simulink model "MG_sim"  (R2020a)
settings: Solver=VariableStepAuto  StartTime=0.0  StopTime=Inf  FixedStep=N*T  RelTol=1e-3
PostLoadFcn:
  | , if any(exist('dsrtsu_mdlpostloadfcn', 'file') ~= 0), dsrtsu_mdlpostloadfcn('Execute', bdroot); end,
InitFcn:
  | , if any(exist('rtifpga_mdlclblib', 'file') ~= 0), rtifpga_mdlclblib('Init', bdroot); end,
model workspace (MAT data in the model file):
  FPGA_MG_sim_1_Register_1_1_1_write : Simulink.Signal (value not decoded)
  FPGA_MG_sim_1_Register_2_1_1_write : Simulink.Signal (value not decoded)
  FPGA_MG_sim_1_Register_3_1_1_write : Simulink.Signal (value not decoded)
values from neighbouring files (symbols this model uses):
  amp = 1    [param.m]
  fixedgain_i = 10*1000/(3*100)    (= 33.3333333333)    [param.m]
  fixedgain_vc1 = 10*10000/(3*100*2.5)    (= 133.333333333)    [param.m]
  fixedgain_vc5 = 10*22000/(3*100*2.5)    (= 293.333333333)    [param.m]
  fixedgain_vdc = 10*22000/(3*100*2.5)    (= 293.333333333)    [param.m]
  freq = 50    [param.m]
  gain_iL1 = 1    [param.m]
  gain_iL2 = 1    [param.m]
  gain_iL3 = 1    [param.m]
  gain_iL4 = 1    [param.m]
  gain_vc1 = 1    [param.m]
  gain_vc5 = 1    [param.m]
  gain_vdc = 1    [param.m]
  Ii = 10    [param.m]
  Ipv = 0.01    [param.m]
  Iv = 0.1    [param.m]
  Ki = 1e-7    (= 1e-07)    [param.m]
  Kp = 0.5    [param.m]
  M = 10    [param.m]
  maxd = N-1    (= 39)    [param.m]
  mind = 1    [param.m]
  N = 40    [param.m]
  offset_iL1 = .2    (= 0.2)    [param.m]
  offset_iL2 = 0.2    [param.m]
  offset_iL3 = 0.3    [param.m]
  offset_iL4 = 0.25    [param.m]
  offset_vc1 = 0.27    [param.m]
  offset_vc5 = 1.3    [param.m]
  offset_vdc = 1.5    [param.m]
  Pi = 0.3    [param.m]
  Ppv = 0.05    [param.m]
  Pv = 0.05    [param.m]
  T = 6e-6    (= 6e-06)    [param.m]
  Tf = 1/1000    (= 0.001)    [param.m]
  Tfdc = 1/20    (= 0.05)    [param.m]
  v_dc_ref = 80    [param.m]
undefined symbols (not defined in the file or in its folder): DiscIntNeverNeededParam
libraries: xbsIndex_r4 x156, rti1202lib_adc_class1 x7, rtiproclib x7, simulink x6, rti1202lib_dac_class1 x1, rtifpgainterfacelib x1
(part 4 of 5)

== system MG_sim/RTI Data/RTI Data Store ==
  RTI Data Store : Subsystem  mask(RTI_DATA_STORE){}
      mask help:
      | RTI Data Store Block. This block is used by RTI to store internal model dependent data. Deleting this block will result in data loss.
      |
      | NEVER DELETE, COPY, OR MODIFY THIS BLOCK!
      mask Help:
      | RTI Data Store Block. This block is used by RTI to store internal model dependent data. Deleting this block will result in data loss.
      | 
      | NEVER DELETE, COPY, OR MODIFY THIS BLOCK!
      mask Display: text(0.5, 0.5, ' ', 'HorizontalAlignment', 'center');

== system MG_sim/fpga/FPGA_INT_BL1 ==
  Int : Inport
  CEP1 : xbsIndex_r4/Clock Enable Probe  inherit_constraints=off  block_type=ceprobe
      settings: infoedit="Clock enable extractor.  Produces a Boolean output that mirrors the hardware clock enable associated with the input sample rate.<br><br>Hardware notes: in hardware this block costs nothing."
  Constant1 : xbsIndex_r4/Constant  const=1  gui_display_data_type=Fixed-point  arith_type=Boolean  n_bits=16  bin_pt=14  preci_type=Single  exp_width=8  frac_width=24  explicit_period=on  period=1*1e-08  equ=P=C  opselect=C  inp2=PCIN>>17  opr=+  inp1=P  carry=CIN  dbl_ovrd=off  block_type=constant
  Convert1 : xbsIndex_r4/Convert  gui_display_data_type=Fixed-point  arith_type=Unsigned  n_bits=1  bin_pt=0  float_type=Single  exp_bits=8  fraction_bits=24  quantization=Truncate  overflow=Wrap  en=off  latency=0  pipeline=off  dbl_ovrd=off  block_type=convert
  Register1 : xbsIndex_r4/Register  init=0  rst=off  en=on  dbl_ovrd=off  block_type=register
  Terminator : Terminator
  phs_interrupt : Subsystem
  usr_interrupt_02 : xbsIndex_r4/Gateway Out  inherit_from_input=off  hdl_port=on  rows=1  columns=1  UseAsDAC=off  DACChannel='1'  interface=None  automatic_assignment=on  address_offset=hex2dec('00')  intf_name=''  intf_description=''  timing_constraint=None  locs_specified=off  LOCs={}  io_standard={}  block_type=gatewayout
  tag scope: FPGA_MG_sim_rtiFPGAtmp_1_Interrupt_3_1_write=global
  wires:
  phs_interrupt/1(data_o) -> [FPGA_MG_sim_rtiFPGAtmp_1_Interrupt_3_1_write], Terminator/1
  usr_interrupt_02/1 -> phs_interrupt/1(data_i)
  Convert1/1 -> Register1/1
  Int/1 -> Convert1/1
  Register1/1 -> usr_interrupt_02/1
  CEP1/1 -> Register1/2
  Constant1/1 -> CEP1/1

== system MG_sim/fpga/FPGA_INT_BL2 ==
  Int : Inport
  CEP1 : xbsIndex_r4/Clock Enable Probe  inherit_constraints=off  block_type=ceprobe
      settings: infoedit="Clock enable extractor.  Produces a Boolean output that mirrors the hardware clock enable associated with the input sample rate.<br><br>Hardware notes: in hardware this block costs nothing."
  Constant1 : xbsIndex_r4/Constant  const=1  gui_display_data_type=Fixed-point  arith_type=Boolean  n_bits=16  bin_pt=14  preci_type=Single  exp_width=8  frac_width=24  explicit_period=on  period=1*1e-08  equ=P=C  opselect=C  inp2=PCIN>>17  opr=+  inp1=P  carry=CIN  dbl_ovrd=off  block_type=constant
  Convert1 : xbsIndex_r4/Convert  gui_display_data_type=Fixed-point  arith_type=Unsigned  n_bits=1  bin_pt=0  float_type=Single  exp_bits=8  fraction_bits=24  quantization=Truncate  overflow=Wrap  en=off  latency=0  pipeline=off  dbl_ovrd=off  block_type=convert
  Register1 : xbsIndex_r4/Register  init=0  rst=off  en=on  dbl_ovrd=off  block_type=register
  Terminator : Terminator
  phs_interrupt : Subsystem
  usr_interrupt_01 : xbsIndex_r4/Gateway Out  inherit_from_input=off  hdl_port=on  rows=1  columns=1  UseAsDAC=off  DACChannel='1'  interface=None  automatic_assignment=on  address_offset=hex2dec('00')  intf_name=''  intf_description=''  timing_constraint=None  locs_specified=off  LOCs={}  io_standard={}  block_type=gatewayout
  tag scope: FPGA_MG_sim_rtiFPGAtmp_1_Interrupt_2_1_write=global
  wires:
  phs_interrupt/1(data_o) -> [FPGA_MG_sim_rtiFPGAtmp_1_Interrupt_2_1_write], Terminator/1
  usr_interrupt_01/1 -> phs_interrupt/1(data_i)
  Convert1/1 -> Register1/1
  Int/1 -> Convert1/1
  Register1/1 -> usr_interrupt_01/1
  CEP1/1 -> Register1/2
  Constant1/1 -> CEP1/1

== system MG_sim/fpga/FPGA_INT_BL3 ==
  Int : Inport
  CEP1 : xbsIndex_r4/Clock Enable Probe  inherit_constraints=off  block_type=ceprobe
      settings: infoedit="Clock enable extractor.  Produces a Boolean output that mirrors the hardware clock enable associated with the input sample rate.<br><br>Hardware notes: in hardware this block costs nothing."
  Constant1 : xbsIndex_r4/Constant  const=1  gui_display_data_type=Fixed-point  arith_type=Boolean  n_bits=16  bin_pt=14  preci_type=Single  exp_width=8  frac_width=24  explicit_period=on  period=1*1e-08  equ=P=C  opselect=C  inp2=PCIN>>17  opr=+  inp1=P  carry=CIN  dbl_ovrd=off  block_type=constant
  Convert1 : xbsIndex_r4/Convert  gui_display_data_type=Fixed-point  arith_type=Unsigned  n_bits=1  bin_pt=0  float_type=Single  exp_bits=8  fraction_bits=24  quantization=Truncate  overflow=Wrap  en=off  latency=0  pipeline=off  dbl_ovrd=off  block_type=convert
  Register1 : xbsIndex_r4/Register  init=0  rst=off  en=on  dbl_ovrd=off  block_type=register
  Terminator : Terminator
  phs_interrupt : Subsystem
  usr_interrupt_00 : xbsIndex_r4/Gateway Out  inherit_from_input=off  hdl_port=on  rows=1  columns=1  UseAsDAC=off  DACChannel='1'  interface=None  automatic_assignment=on  address_offset=hex2dec('00')  intf_name=''  intf_description=''  timing_constraint=None  locs_specified=off  LOCs={}  io_standard={}  block_type=gatewayout
  tag scope: FPGA_MG_sim_rtiFPGAtmp_1_Interrupt_1_1_write=global
  wires:
  phs_interrupt/1(data_o) -> [FPGA_MG_sim_rtiFPGAtmp_1_Interrupt_1_1_write], Terminator/1
  usr_interrupt_00/1 -> phs_interrupt/1(data_i)
  Convert1/1 -> Register1/1
  Int/1 -> Convert1/1
  Register1/1 -> usr_interrupt_00/1
  CEP1/1 -> Register1/2
  Constant1/1 -> CEP1/1

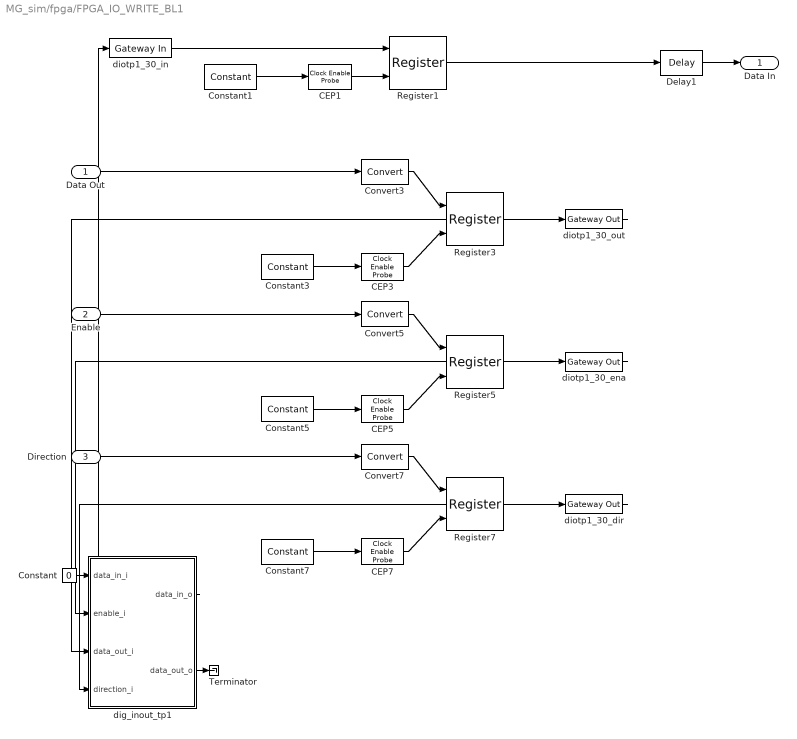
== system MG_sim/fpga/FPGA_IO_WRITE_BL1 ==
  Data Out : Inport
  Enable : Inport  Port=2
  Direction : Inport  Port=3
  CEP{1,3,5,7} (4 alike) : xbsIndex_r4/Clock Enable Probe  inherit_constraints=off  block_type=ceprobe
      settings: infoedit="Clock enable extractor.  Produces a Boolean output that mirrors the hardware clock enable associated with the input sample rate.<br><br>Hardware notes: in hardware this block costs nothing."
  Constant : Constant  Value=0
  Constant{1,3,5,7} (4 alike) : xbsIndex_r4/Constant  const=1  gui_display_data_type=Fixed-point  arith_type=Boolean  n_bits=16  bin_pt=14  preci_type=Single  exp_width=8  frac_width=24  explicit_period=on  period=1*1e-08  equ=P=C  opselect=C  inp2=PCIN>>17  opr=+  inp1=P  carry=CIN  dbl_ovrd=off  block_type=constant
  Convert3 : xbsIndex_r4/Convert  gui_display_data_type=Fixed-point  arith_type=Unsigned  n_bits=1  bin_pt=0  float_type=Single  exp_bits=8  fraction_bits=24  quantization=Truncate  overflow=Wrap  en=off  latency=0  pipeline=off  dbl_ovrd=off  block_type=convert
  Convert5 : xbsIndex_r4/Convert  gui_display_data_type=Fixed-point  arith_type=Unsigned  n_bits=1  bin_pt=0  float_type=Single  exp_bits=8  fraction_bits=24  quantization=Truncate  overflow=Wrap  en=off  latency=0  pipeline=off  dbl_ovrd=off  block_type=convert
  Convert7 : xbsIndex_r4/Convert  gui_display_data_type=Fixed-point  arith_type=Unsigned  n_bits=1  bin_pt=0  float_type=Single  exp_bits=8  fraction_bits=24  quantization=Truncate  overflow=Wrap  en=off  latency=0  pipeline=off  dbl_ovrd=off  block_type=convert
  Delay1 : xbsIndex_r4/Delay  rst=off  infoeditControl=Selection of Reset will increase slice count due to use of real FFs and instead of SRLs  en=off  latency=0  reg_retiming=off  dbl_ovrd=off  block_type=delay
  Register{1,3,5,7} (4 alike) : xbsIndex_r4/Register  init=0  rst=off  en=on  dbl_ovrd=off  block_type=register
  Terminator : Terminator
  dig_inout_tp1 : Subsystem
      mask init:
      | par = rtifpgafcnlib('GetCurrentParaValue', get_param(get(gcbh, 'parent'), 'handle'));
      | if isempty(par)
      |     return
      | end
      | inverted_dio = str2double(par(2).Value{1});
      | vsetting = str2double(par(5).Value{1});
      | switch vsetting 
      |     case 1
      |         voltage = 3.3
      |     case 2
      |         voltage = 2.5;
      |     otherwise
      |         voltage = 5;
      | end
  diotp1_30_dir : xbsIndex_r4/Gateway Out  inherit_from_input=off  hdl_port=on  rows=1  columns=1  UseAsDAC=off  DACChannel='1'  interface=None  automatic_assignment=on  address_offset=hex2dec('00')  intf_name=''  intf_description=''  timing_constraint=None  locs_specified=off  LOCs={}  io_standard={}  block_type=gatewayout
  diotp1_30_ena : xbsIndex_r4/Gateway Out  inherit_from_input=off  hdl_port=on  rows=1  columns=1  UseAsDAC=off  DACChannel='1'  interface=None  automatic_assignment=on  address_offset=hex2dec('00')  intf_name=''  intf_description=''  timing_constraint=None  locs_specified=off  LOCs={}  io_standard={}  block_type=gatewayout
  diotp1_30_in : xbsIndex_r4/Gateway In  gui_display_data_type=Fixed-point  arith_type=Unsigned  n_bits=1  bin_pt=0  preci_type=Single  exp_width=8  frac_width=24  rows=1  columns=1  quantization="Round  (unbiased: +/- Inf)"  overflow=Saturate  period=1e-08  UseAsADC=off  ADCChannel='1'  interface=None  automatic_assignment=on  address_offset=hex2dec('00')  intf_name=''  intf_description=''  default_value=0  timing_constraint=None  locs_specified=off  LOCs={}  io_standard={}  inherit_from_input=off  hdl_port=on  dbl_ovrd=off  block_type=gatewayin
  diotp1_30_out : xbsIndex_r4/Gateway Out  inherit_from_input=off  hdl_port=on  rows=1  columns=1  UseAsDAC=off  DACChannel='1'  interface=None  automatic_assignment=on  address_offset=hex2dec('00')  intf_name=''  intf_description=''  timing_constraint=None  locs_specified=off  LOCs={}  io_standard={}  block_type=gatewayout
  Data In : Outport
  wires:
  dig_inout_tp1/2(data_out_o) -> Terminator/1
  Constant/1 -> dig_inout_tp1/1(data_in_i)
  diotp1_30_dir/1 -> dig_inout_tp1/4(direction_i)
  diotp1_30_ena/1 -> dig_inout_tp1/2(enable_i)
  diotp1_30_out/1 -> dig_inout_tp1/3(data_out_i)
  dig_inout_tp1/1(data_in_o) -> diotp1_30_in/1
  Convert7/1 -> Register7/1
  Direction/1 -> Convert7/1
  Register7/1 -> diotp1_30_dir/1
  CEP7/1 -> Register7/2
  Constant7/1 -> CEP7/1
  Convert5/1 -> Register5/1
  Enable/1 -> Convert5/1
  Register5/1 -> diotp1_30_ena/1
  CEP5/1 -> Register5/2
  Constant5/1 -> CEP5/1
  Convert3/1 -> Register3/1
  Data Out/1 -> Convert3/1
  Register3/1 -> diotp1_30_out/1
  CEP3/1 -> Register3/2
  Constant3/1 -> CEP3/1
  diotp1_30_in/1 -> Register1/1
  CEP1/1 -> Register1/2
  Constant1/1 -> CEP1/1
  Delay1/1 -> Data In/1
  Register1/1 -> Delay1/1

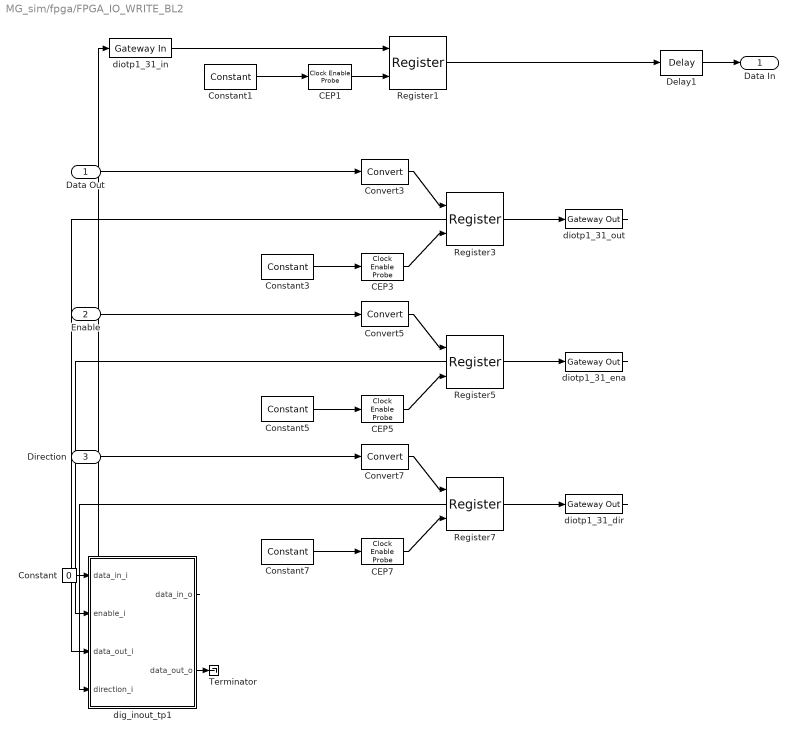
== system MG_sim/fpga/FPGA_IO_WRITE_BL2 ==
  Data Out : Inport
  Enable : Inport  Port=2
  Direction : Inport  Port=3
  CEP{1,3,5,7} (4 alike) : xbsIndex_r4/Clock Enable Probe  inherit_constraints=off  block_type=ceprobe
      settings: infoedit="Clock enable extractor.  Produces a Boolean output that mirrors the hardware clock enable associated with the input sample rate.<br><br>Hardware notes: in hardware this block costs nothing."
  Constant : Constant  Value=0
  Constant{1,3,5,7} (4 alike) : xbsIndex_r4/Constant  const=1  gui_display_data_type=Fixed-point  arith_type=Boolean  n_bits=16  bin_pt=14  preci_type=Single  exp_width=8  frac_width=24  explicit_period=on  period=1*1e-08  equ=P=C  opselect=C  inp2=PCIN>>17  opr=+  inp1=P  carry=CIN  dbl_ovrd=off  block_type=constant
  Convert3 : xbsIndex_r4/Convert  gui_display_data_type=Fixed-point  arith_type=Unsigned  n_bits=1  bin_pt=0  float_type=Single  exp_bits=8  fraction_bits=24  quantization=Truncate  overflow=Wrap  en=off  latency=0  pipeline=off  dbl_ovrd=off  block_type=convert
  Convert5 : xbsIndex_r4/Convert  gui_display_data_type=Fixed-point  arith_type=Unsigned  n_bits=1  bin_pt=0  float_type=Single  exp_bits=8  fraction_bits=24  quantization=Truncate  overflow=Wrap  en=off  latency=0  pipeline=off  dbl_ovrd=off  block_type=convert
  Convert7 : xbsIndex_r4/Convert  gui_display_data_type=Fixed-point  arith_type=Unsigned  n_bits=1  bin_pt=0  float_type=Single  exp_bits=8  fraction_bits=24  quantization=Truncate  overflow=Wrap  en=off  latency=0  pipeline=off  dbl_ovrd=off  block_type=convert
  Delay1 : xbsIndex_r4/Delay  rst=off  infoeditControl=Selection of Reset will increase slice count due to use of real FFs and instead of SRLs  en=off  latency=0  reg_retiming=off  dbl_ovrd=off  block_type=delay
  Register{1,3,5,7} (4 alike) : xbsIndex_r4/Register  init=0  rst=off  en=on  dbl_ovrd=off  block_type=register
  Terminator : Terminator
  dig_inout_tp1 : Subsystem
      mask init: same as MG_sim/fpga/FPGA_IO_WRITE_BL1/dig_inout_tp1
  diotp1_31_dir : xbsIndex_r4/Gateway Out  inherit_from_input=off  hdl_port=on  rows=1  columns=1  UseAsDAC=off  DACChannel='1'  interface=None  automatic_assignment=on  address_offset=hex2dec('00')  intf_name=''  intf_description=''  timing_constraint=None  locs_specified=off  LOCs={}  io_standard={}  block_type=gatewayout
  diotp1_31_ena : xbsIndex_r4/Gateway Out  inherit_from_input=off  hdl_port=on  rows=1  columns=1  UseAsDAC=off  DACChannel='1'  interface=None  automatic_assignment=on  address_offset=hex2dec('00')  intf_name=''  intf_description=''  timing_constraint=None  locs_specified=off  LOCs={}  io_standard={}  block_type=gatewayout
  diotp1_31_in : xbsIndex_r4/Gateway In  gui_display_data_type=Fixed-point  arith_type=Unsigned  n_bits=1  bin_pt=0  preci_type=Single  exp_width=8  frac_width=24  rows=1  columns=1  quantization="Round  (unbiased: +/- Inf)"  overflow=Saturate  period=1e-08  UseAsADC=off  ADCChannel='1'  interface=None  automatic_assignment=on  address_offset=hex2dec('00')  intf_name=''  intf_description=''  default_value=0  timing_constraint=None  locs_specified=off  LOCs={}  io_standard={}  inherit_from_input=off  hdl_port=on  dbl_ovrd=off  block_type=gatewayin
  diotp1_31_out : xbsIndex_r4/Gateway Out  inherit_from_input=off  hdl_port=on  rows=1  columns=1  UseAsDAC=off  DACChannel='1'  interface=None  automatic_assignment=on  address_offset=hex2dec('00')  intf_name=''  intf_description=''  timing_constraint=None  locs_specified=off  LOCs={}  io_standard={}  block_type=gatewayout
  Data In : Outport
  wires:
  dig_inout_tp1/2(data_out_o) -> Terminator/1
  Constant/1 -> dig_inout_tp1/1(data_in_i)
  diotp1_31_dir/1 -> dig_inout_tp1/4(direction_i)
  diotp1_31_ena/1 -> dig_inout_tp1/2(enable_i)
  diotp1_31_out/1 -> dig_inout_tp1/3(data_out_i)
  dig_inout_tp1/1(data_in_o) -> diotp1_31_in/1
  Convert7/1 -> Register7/1
  Direction/1 -> Convert7/1
  Register7/1 -> diotp1_31_dir/1
  CEP7/1 -> Register7/2
  Constant7/1 -> CEP7/1
  Convert5/1 -> Register5/1
  Enable/1 -> Convert5/1
  Register5/1 -> diotp1_31_ena/1
  CEP5/1 -> Register5/2
  Constant5/1 -> CEP5/1
  Convert3/1 -> Register3/1
  Data Out/1 -> Convert3/1
  Register3/1 -> diotp1_31_out/1
  CEP3/1 -> Register3/2
  Constant3/1 -> CEP3/1
  diotp1_31_in/1 -> Register1/1
  CEP1/1 -> Register1/2
  Constant1/1 -> CEP1/1
  Delay1/1 -> Data In/1
  Register1/1 -> Delay1/1

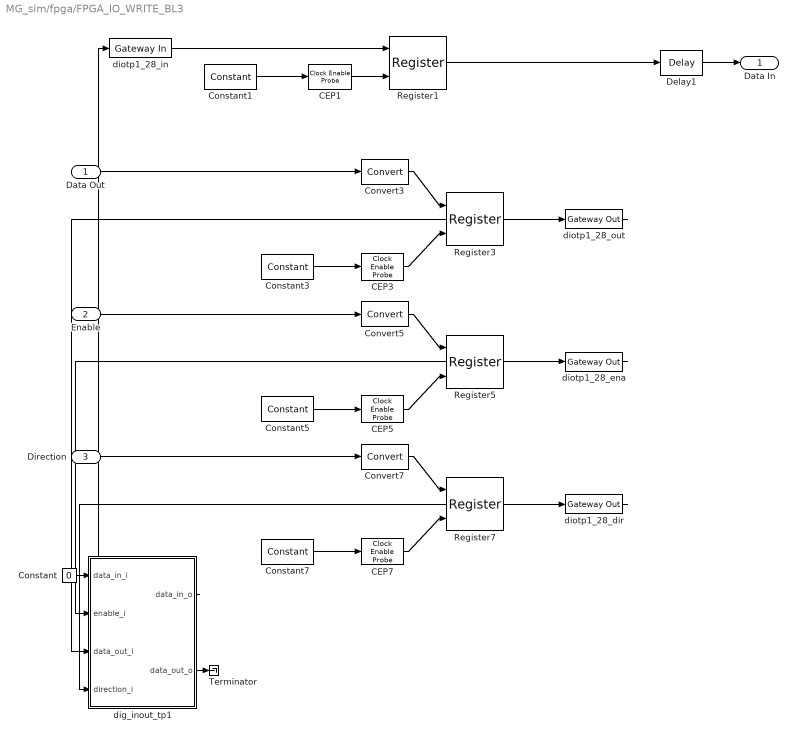
== system MG_sim/fpga/FPGA_IO_WRITE_BL3 ==
  Data Out : Inport
  Enable : Inport  Port=2
  Direction : Inport  Port=3
  CEP{1,3,5,7} (4 alike) : xbsIndex_r4/Clock Enable Probe  inherit_constraints=off  block_type=ceprobe
      settings: infoedit="Clock enable extractor.  Produces a Boolean output that mirrors the hardware clock enable associated with the input sample rate.<br><br>Hardware notes: in hardware this block costs nothing."
  Constant : Constant  Value=0
  Constant{1,3,5,7} (4 alike) : xbsIndex_r4/Constant  const=1  gui_display_data_type=Fixed-point  arith_type=Boolean  n_bits=16  bin_pt=14  preci_type=Single  exp_width=8  frac_width=24  explicit_period=on  period=1*1e-08  equ=P=C  opselect=C  inp2=PCIN>>17  opr=+  inp1=P  carry=CIN  dbl_ovrd=off  block_type=constant
  Convert3 : xbsIndex_r4/Convert  gui_display_data_type=Fixed-point  arith_type=Unsigned  n_bits=1  bin_pt=0  float_type=Single  exp_bits=8  fraction_bits=24  quantization=Truncate  overflow=Wrap  en=off  latency=0  pipeline=off  dbl_ovrd=off  block_type=convert
  Convert5 : xbsIndex_r4/Convert  gui_display_data_type=Fixed-point  arith_type=Unsigned  n_bits=1  bin_pt=0  float_type=Single  exp_bits=8  fraction_bits=24  quantization=Truncate  overflow=Wrap  en=off  latency=0  pipeline=off  dbl_ovrd=off  block_type=convert
  Convert7 : xbsIndex_r4/Convert  gui_display_data_type=Fixed-point  arith_type=Unsigned  n_bits=1  bin_pt=0  float_type=Single  exp_bits=8  fraction_bits=24  quantization=Truncate  overflow=Wrap  en=off  latency=0  pipeline=off  dbl_ovrd=off  block_type=convert
  Delay1 : xbsIndex_r4/Delay  rst=off  infoeditControl=Selection of Reset will increase slice count due to use of real FFs and instead of SRLs  en=off  latency=0  reg_retiming=off  dbl_ovrd=off  block_type=delay
  Register{1,3,5,7} (4 alike) : xbsIndex_r4/Register  init=0  rst=off  en=on  dbl_ovrd=off  block_type=register
  Terminator : Terminator
  dig_inout_tp1 : Subsystem
      mask init: same as MG_sim/fpga/FPGA_IO_WRITE_BL1/dig_inout_tp1
  diotp1_28_dir : xbsIndex_r4/Gateway Out  inherit_from_input=off  hdl_port=on  rows=1  columns=1  UseAsDAC=off  DACChannel='1'  interface=None  automatic_assignment=on  address_offset=hex2dec('00')  intf_name=''  intf_description=''  timing_constraint=None  locs_specified=off  LOCs={}  io_standard={}  block_type=gatewayout
  diotp1_28_ena : xbsIndex_r4/Gateway Out  inherit_from_input=off  hdl_port=on  rows=1  columns=1  UseAsDAC=off  DACChannel='1'  interface=None  automatic_assignment=on  address_offset=hex2dec('00')  intf_name=''  intf_description=''  timing_constraint=None  locs_specified=off  LOCs={}  io_standard={}  block_type=gatewayout
  diotp1_28_in : xbsIndex_r4/Gateway In  gui_display_data_type=Fixed-point  arith_type=Unsigned  n_bits=1  bin_pt=0  preci_type=Single  exp_width=8  frac_width=24  rows=1  columns=1  quantization="Round  (unbiased: +/- Inf)"  overflow=Saturate  period=1e-08  UseAsADC=off  ADCChannel='1'  interface=None  automatic_assignment=on  address_offset=hex2dec('00')  intf_name=''  intf_description=''  default_value=0  timing_constraint=None  locs_specified=off  LOCs={}  io_standard={}  inherit_from_input=off  hdl_port=on  dbl_ovrd=off  block_type=gatewayin
  diotp1_28_out : xbsIndex_r4/Gateway Out  inherit_from_input=off  hdl_port=on  rows=1  columns=1  UseAsDAC=off  DACChannel='1'  interface=None  automatic_assignment=on  address_offset=hex2dec('00')  intf_name=''  intf_description=''  timing_constraint=None  locs_specified=off  LOCs={}  io_standard={}  block_type=gatewayout
  Data In : Outport
  wires:
  dig_inout_tp1/2(data_out_o) -> Terminator/1
  Constant/1 -> dig_inout_tp1/1(data_in_i)
  diotp1_28_dir/1 -> dig_inout_tp1/4(direction_i)
  diotp1_28_ena/1 -> dig_inout_tp1/2(enable_i)
  diotp1_28_out/1 -> dig_inout_tp1/3(data_out_i)
  dig_inout_tp1/1(data_in_o) -> diotp1_28_in/1
  Convert7/1 -> Register7/1
  Direction/1 -> Convert7/1
  Register7/1 -> diotp1_28_dir/1
  CEP7/1 -> Register7/2
  Constant7/1 -> CEP7/1
  Convert5/1 -> Register5/1
  Enable/1 -> Convert5/1
  Register5/1 -> diotp1_28_ena/1
  CEP5/1 -> Register5/2
  Constant5/1 -> CEP5/1
  Convert3/1 -> Register3/1
  Data Out/1 -> Convert3/1
  Register3/1 -> diotp1_28_out/1
  CEP3/1 -> Register3/2
  Constant3/1 -> CEP3/1
  diotp1_28_in/1 -> Register1/1
  CEP1/1 -> Register1/2
  Constant1/1 -> CEP1/1
  Delay1/1 -> Data In/1
  Register1/1 -> Delay1/1

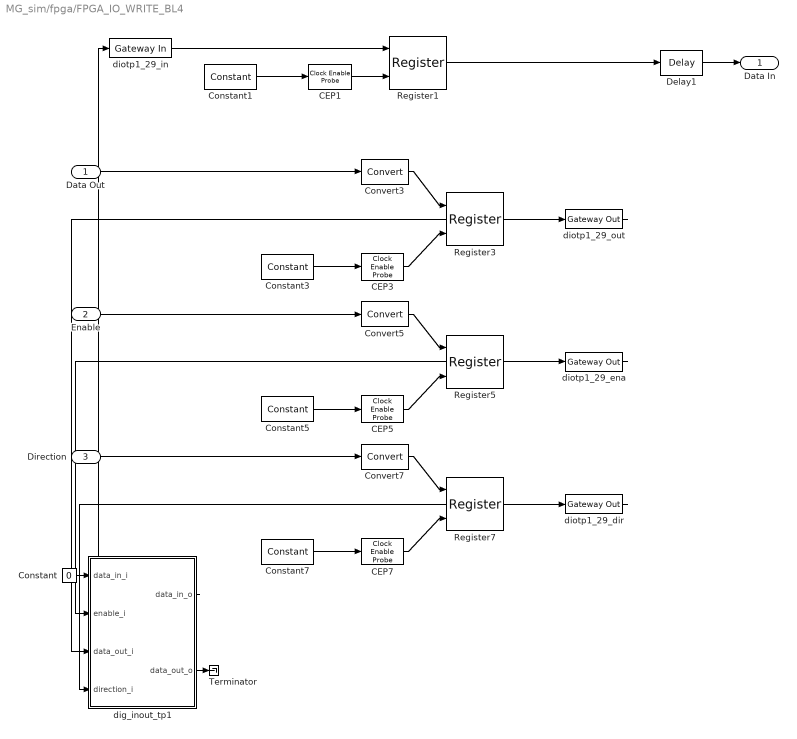
== system MG_sim/fpga/FPGA_IO_WRITE_BL4 ==
  Data Out : Inport
  Enable : Inport  Port=2
  Direction : Inport  Port=3
  CEP{1,3,5,7} (4 alike) : xbsIndex_r4/Clock Enable Probe  inherit_constraints=off  block_type=ceprobe
      settings: infoedit="Clock enable extractor.  Produces a Boolean output that mirrors the hardware clock enable associated with the input sample rate.<br><br>Hardware notes: in hardware this block costs nothing."
  Constant : Constant  Value=0
  Constant{1,3,5,7} (4 alike) : xbsIndex_r4/Constant  const=1  gui_display_data_type=Fixed-point  arith_type=Boolean  n_bits=16  bin_pt=14  preci_type=Single  exp_width=8  frac_width=24  explicit_period=on  period=1*1e-08  equ=P=C  opselect=C  inp2=PCIN>>17  opr=+  inp1=P  carry=CIN  dbl_ovrd=off  block_type=constant
  Convert3 : xbsIndex_r4/Convert  gui_display_data_type=Fixed-point  arith_type=Unsigned  n_bits=1  bin_pt=0  float_type=Single  exp_bits=8  fraction_bits=24  quantization=Truncate  overflow=Wrap  en=off  latency=0  pipeline=off  dbl_ovrd=off  block_type=convert
  Convert5 : xbsIndex_r4/Convert  gui_display_data_type=Fixed-point  arith_type=Unsigned  n_bits=1  bin_pt=0  float_type=Single  exp_bits=8  fraction_bits=24  quantization=Truncate  overflow=Wrap  en=off  latency=0  pipeline=off  dbl_ovrd=off  block_type=convert
  Convert7 : xbsIndex_r4/Convert  gui_display_data_type=Fixed-point  arith_type=Unsigned  n_bits=1  bin_pt=0  float_type=Single  exp_bits=8  fraction_bits=24  quantization=Truncate  overflow=Wrap  en=off  latency=0  pipeline=off  dbl_ovrd=off  block_type=convert
  Delay1 : xbsIndex_r4/Delay  rst=off  infoeditControl=Selection of Reset will increase slice count due to use of real FFs and instead of SRLs  en=off  latency=0  reg_retiming=off  dbl_ovrd=off  block_type=delay
  Register{1,3,5,7} (4 alike) : xbsIndex_r4/Register  init=0  rst=off  en=on  dbl_ovrd=off  block_type=register
  Terminator : Terminator
  dig_inout_tp1 : Subsystem
      mask init: same as MG_sim/fpga/FPGA_IO_WRITE_BL1/dig_inout_tp1
  diotp1_29_dir : xbsIndex_r4/Gateway Out  inherit_from_input=off  hdl_port=on  rows=1  columns=1  UseAsDAC=off  DACChannel='1'  interface=None  automatic_assignment=on  address_offset=hex2dec('00')  intf_name=''  intf_description=''  timing_constraint=None  locs_specified=off  LOCs={}  io_standard={}  block_type=gatewayout
  diotp1_29_ena : xbsIndex_r4/Gateway Out  inherit_from_input=off  hdl_port=on  rows=1  columns=1  UseAsDAC=off  DACChannel='1'  interface=None  automatic_assignment=on  address_offset=hex2dec('00')  intf_name=''  intf_description=''  timing_constraint=None  locs_specified=off  LOCs={}  io_standard={}  block_type=gatewayout
  diotp1_29_in : xbsIndex_r4/Gateway In  gui_display_data_type=Fixed-point  arith_type=Unsigned  n_bits=1  bin_pt=0  preci_type=Single  exp_width=8  frac_width=24  rows=1  columns=1  quantization="Round  (unbiased: +/- Inf)"  overflow=Saturate  period=1e-08  UseAsADC=off  ADCChannel='1'  interface=None  automatic_assignment=on  address_offset=hex2dec('00')  intf_name=''  intf_description=''  default_value=0  timing_constraint=None  locs_specified=off  LOCs={}  io_standard={}  inherit_from_input=off  hdl_port=on  dbl_ovrd=off  block_type=gatewayin
  diotp1_29_out : xbsIndex_r4/Gateway Out  inherit_from_input=off  hdl_port=on  rows=1  columns=1  UseAsDAC=off  DACChannel='1'  interface=None  automatic_assignment=on  address_offset=hex2dec('00')  intf_name=''  intf_description=''  timing_constraint=None  locs_specified=off  LOCs={}  io_standard={}  block_type=gatewayout
  Data In : Outport
  wires:
  dig_inout_tp1/2(data_out_o) -> Terminator/1
  Constant/1 -> dig_inout_tp1/1(data_in_i)
  diotp1_29_dir/1 -> dig_inout_tp1/4(direction_i)
  diotp1_29_ena/1 -> dig_inout_tp1/2(enable_i)
  diotp1_29_out/1 -> dig_inout_tp1/3(data_out_i)
  dig_inout_tp1/1(data_in_o) -> diotp1_29_in/1
  Convert7/1 -> Register7/1
  Direction/1 -> Convert7/1
  Register7/1 -> diotp1_29_dir/1
  CEP7/1 -> Register7/2
  Constant7/1 -> CEP7/1
  Convert5/1 -> Register5/1
  Enable/1 -> Convert5/1
  Register5/1 -> diotp1_29_ena/1
  CEP5/1 -> Register5/2
  Constant5/1 -> CEP5/1
  Convert3/1 -> Register3/1
  Data Out/1 -> Convert3/1
  Register3/1 -> diotp1_29_out/1
  CEP3/1 -> Register3/2
  Constant3/1 -> CEP3/1
  diotp1_29_in/1 -> Register1/1
  CEP1/1 -> Register1/2
  Constant1/1 -> CEP1/1
  Delay1/1 -> Data In/1
  Register1/1 -> Delay1/1

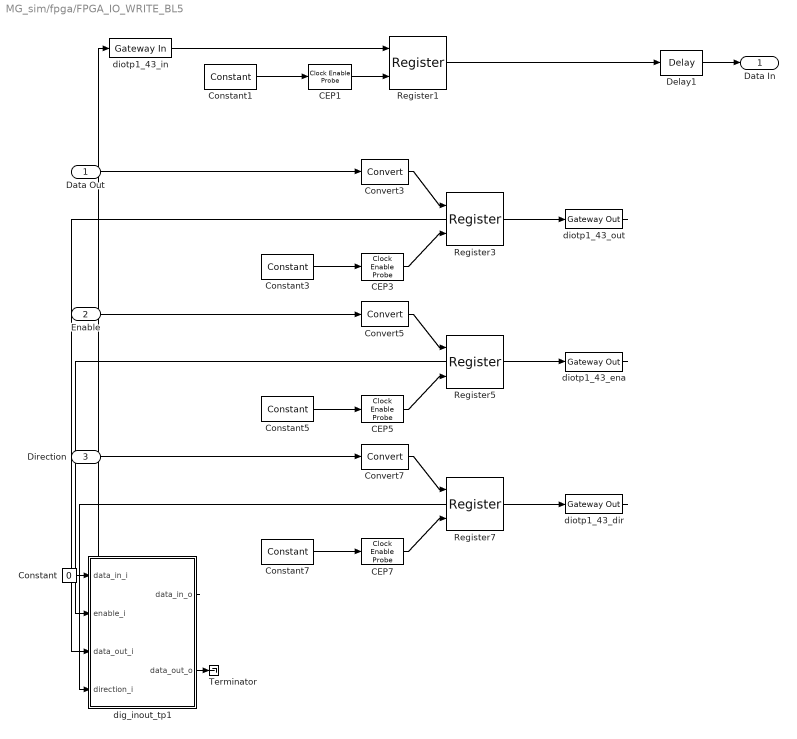
== system MG_sim/fpga/FPGA_IO_WRITE_BL5 ==
  Data Out : Inport
  Enable : Inport  Port=2
  Direction : Inport  Port=3
  CEP{1,3,5,7} (4 alike) : xbsIndex_r4/Clock Enable Probe  inherit_constraints=off  block_type=ceprobe
      settings: infoedit="Clock enable extractor.  Produces a Boolean output that mirrors the hardware clock enable associated with the input sample rate.<br><br>Hardware notes: in hardware this block costs nothing."
  Constant : Constant  Value=0
  Constant{1,3,5,7} (4 alike) : xbsIndex_r4/Constant  const=1  gui_display_data_type=Fixed-point  arith_type=Boolean  n_bits=16  bin_pt=14  preci_type=Single  exp_width=8  frac_width=24  explicit_period=on  period=1*1e-08  equ=P=C  opselect=C  inp2=PCIN>>17  opr=+  inp1=P  carry=CIN  dbl_ovrd=off  block_type=constant
  Convert3 : xbsIndex_r4/Convert  gui_display_data_type=Fixed-point  arith_type=Unsigned  n_bits=1  bin_pt=0  float_type=Single  exp_bits=8  fraction_bits=24  quantization=Truncate  overflow=Wrap  en=off  latency=0  pipeline=off  dbl_ovrd=off  block_type=convert
  Convert5 : xbsIndex_r4/Convert  gui_display_data_type=Fixed-point  arith_type=Unsigned  n_bits=1  bin_pt=0  float_type=Single  exp_bits=8  fraction_bits=24  quantization=Truncate  overflow=Wrap  en=off  latency=0  pipeline=off  dbl_ovrd=off  block_type=convert
  Convert7 : xbsIndex_r4/Convert  gui_display_data_type=Fixed-point  arith_type=Unsigned  n_bits=1  bin_pt=0  float_type=Single  exp_bits=8  fraction_bits=24  quantization=Truncate  overflow=Wrap  en=off  latency=0  pipeline=off  dbl_ovrd=off  block_type=convert
  Delay1 : xbsIndex_r4/Delay  rst=off  infoeditControl=Selection of Reset will increase slice count due to use of real FFs and instead of SRLs  en=off  latency=0  reg_retiming=off  dbl_ovrd=off  block_type=delay
  Register{1,3,5,7} (4 alike) : xbsIndex_r4/Register  init=0  rst=off  en=on  dbl_ovrd=off  block_type=register
  Terminator : Terminator
  dig_inout_tp1 : Subsystem
      mask init: same as MG_sim/fpga/FPGA_IO_WRITE_BL1/dig_inout_tp1
  diotp1_43_dir : xbsIndex_r4/Gateway Out  inherit_from_input=off  hdl_port=on  rows=1  columns=1  UseAsDAC=off  DACChannel='1'  interface=None  automatic_assignment=on  address_offset=hex2dec('00')  intf_name=''  intf_description=''  timing_constraint=None  locs_specified=off  LOCs={}  io_standard={}  block_type=gatewayout
  diotp1_43_ena : xbsIndex_r4/Gateway Out  inherit_from_input=off  hdl_port=on  rows=1  columns=1  UseAsDAC=off  DACChannel='1'  interface=None  automatic_assignment=on  address_offset=hex2dec('00')  intf_name=''  intf_description=''  timing_constraint=None  locs_specified=off  LOCs={}  io_standard={}  block_type=gatewayout
  diotp1_43_in : xbsIndex_r4/Gateway In  gui_display_data_type=Fixed-point  arith_type=Unsigned  n_bits=1  bin_pt=0  preci_type=Single  exp_width=8  frac_width=24  rows=1  columns=1  quantization="Round  (unbiased: +/- Inf)"  overflow=Saturate  period=1e-08  UseAsADC=off  ADCChannel='1'  interface=None  automatic_assignment=on  address_offset=hex2dec('00')  intf_name=''  intf_description=''  default_value=0  timing_constraint=None  locs_specified=off  LOCs={}  io_standard={}  inherit_from_input=off  hdl_port=on  dbl_ovrd=off  block_type=gatewayin
  diotp1_43_out : xbsIndex_r4/Gateway Out  inherit_from_input=off  hdl_port=on  rows=1  columns=1  UseAsDAC=off  DACChannel='1'  interface=None  automatic_assignment=on  address_offset=hex2dec('00')  intf_name=''  intf_description=''  timing_constraint=None  locs_specified=off  LOCs={}  io_standard={}  block_type=gatewayout
  Data In : Outport
  wires:
  dig_inout_tp1/2(data_out_o) -> Terminator/1
  Constant/1 -> dig_inout_tp1/1(data_in_i)
  diotp1_43_dir/1 -> dig_inout_tp1/4(direction_i)
  diotp1_43_ena/1 -> dig_inout_tp1/2(enable_i)
  diotp1_43_out/1 -> dig_inout_tp1/3(data_out_i)
  dig_inout_tp1/1(data_in_o) -> diotp1_43_in/1
  Convert7/1 -> Register7/1
  Direction/1 -> Convert7/1
  Register7/1 -> diotp1_43_dir/1
  CEP7/1 -> Register7/2
  Constant7/1 -> CEP7/1
  Convert5/1 -> Register5/1
  Enable/1 -> Convert5/1
  Register5/1 -> diotp1_43_ena/1
  CEP5/1 -> Register5/2
  Constant5/1 -> CEP5/1
  Convert3/1 -> Register3/1
  Data Out/1 -> Convert3/1
  Register3/1 -> diotp1_43_out/1
  CEP3/1 -> Register3/2
  Constant3/1 -> CEP3/1
  diotp1_43_in/1 -> Register1/1
  CEP1/1 -> Register1/2
  Constant1/1 -> CEP1/1
  Delay1/1 -> Data In/1
  Register1/1 -> Delay1/1

== system MG_sim/fpga/FPGA_XDATA_READ_BL1 ==
  CEP1 : xbsIndex_r4/Clock Enable Probe  inherit_constraints=off  block_type=ceprobe
      settings: infoedit="Clock enable extractor.  Produces a Boolean output that mirrors the hardware clock enable associated with the input sample rate.<br><br>Hardware notes: in hardware this block costs nothing."
  CEP3 : xbsIndex_r4/Clock Enable Probe  inherit_constraints=off  block_type=ceprobe
      settings: infoedit="Clock enable extractor.  Produces a Boolean output that mirrors the hardware clock enable associated with the input sample rate.<br><br>Hardware notes: in hardware this block costs nothing."
  Constant1 : xbsIndex_r4/Constant  const=1  gui_display_data_type=Fixed-point  arith_type=Boolean  n_bits=16  bin_pt=14  preci_type=Single  exp_width=8  frac_width=24  explicit_period=on  period=1*1e-08  equ=P=C  opselect=C  inp2=PCIN>>17  opr=+  inp1=P  carry=CIN  dbl_ovrd=off  block_type=constant
  Constant3 : xbsIndex_r4/Constant  const=1  gui_display_data_type=Fixed-point  arith_type=Boolean  n_bits=16  bin_pt=14  preci_type=Single  exp_width=8  frac_width=24  explicit_period=on  period=1*1e-08  equ=P=C  opselect=C  inp2=PCIN>>17  opr=+  inp1=P  carry=CIN  dbl_ovrd=off  block_type=constant
  Delay1 : xbsIndex_r4/Delay  rst=off  infoeditControl=Selection of Reset will increase slice count due to use of real FFs and instead of SRLs  en=off  latency=0  reg_retiming=off  dbl_ovrd=off  block_type=delay
  Delay3 : xbsIndex_r4/Delay  rst=off  infoeditControl=Selection of Reset will increase slice count due to use of real FFs and instead of SRLs  en=off  latency=0  reg_retiming=off  dbl_ovrd=off  block_type=delay
  Register1 : xbsIndex_r4/Register  init=0  rst=off  en=on  dbl_ovrd=off  block_type=register
  Register3 : xbsIndex_r4/Register  init=0  rst=off  en=on  dbl_ovrd=off  block_type=register
  phs_read_register : Subsystem
      mask init:
      | [par, fct] = rtifpgafcnlib('GetCurrentParaValue', get_param(get(gcbh, 'parent'), 'handle'), 'all');
      | if isempty(par) || isempty(fct)
      |     return
      | end
      | binaryPoint = str2double(par(1).Value{1});
      | format = par(2).Value{1};
      | if (strcmp(format, 'signed') == 1)
      |     mode = 0;
      | elseif (strcmp(format, 'unsigned') == 1)
      |     mode = 1;
      | else
      |     % floating-point
      |     mode = 2;
      | end
      | 
      | %Determine PROC sample time
      | proc_sample_time_field = par(5).Value{1};
      | num_val = str2num(proc_sample_time_field);
      | if ~isempty(num_val)
      |     proc_sample_time = num_val;
      | else % search for subsystem/workspace value
      |     proc_sample_time = rtifpgafcnlib('SearchVariableValue', gcbh, proc_sample_time_field);
      |     if ~isnumeric(proc_sample_time)
      |         proc_sample_time = str2double(proc_sample_time);
      |     end
      | end
      | 
      | %Determine FPGA sample rate
      | dataGatewayName = fct.FrameworkIn(1).Name{1};
      | fpga_sample_time = rtifpga_xsgcasinglib('xlGetParam', [gcs '/' dataGatewayName] , 'period');
      | fpga_sample_time = str2double(fpga_sample_time);
  xreg_000_dout : xbsIndex_r4/Gateway In  gui_display_data_type=Fixed-point  arith_type=Unsigned  n_bits=32  bin_pt=0  preci_type=Single  exp_width=8  frac_width=24  rows=1  columns=1  quantization="Round  (unbiased: +/- Inf)"  overflow=Saturate  period=1e-08  UseAsADC=off  ADCChannel='1'  interface=None  automatic_assignment=on  address_offset=hex2dec('00')  intf_name=''  intf_description=''  default_value=0  timing_constraint=None  locs_specified=off  LOCs={}  io_standard={}  inherit_from_input=off  hdl_port=on  dbl_ovrd=off  block_type=gatewayin
  xreg_000_dout_wr : xbsIndex_r4/Gateway In  gui_display_data_type=Fixed-point  arith_type=Unsigned  n_bits=1  bin_pt=0  preci_type=Single  exp_width=8  frac_width=24  rows=1  columns=1  quantization="Round  (unbiased: +/- Inf)"  overflow=Saturate  period=1e-08  UseAsADC=off  ADCChannel='1'  interface=None  automatic_assignment=on  address_offset=hex2dec('00')  intf_name=''  intf_description=''  default_value=0  timing_constraint=None  locs_specified=off  LOCs={}  io_standard={}  inherit_from_input=off  hdl_port=on  dbl_ovrd=off  block_type=gatewayin
  Data : Outport
  Data New : Outport  Port=2
  wires:
  [FPGA_MG_sim_rtiFPGAtmp_1_Register_1_1_1_write] -> phs_read_register/1(data_i)
  phs_read_register/2(data_new_o) -> xreg_000_dout_wr/1
  phs_read_register/1(data_o) -> xreg_000_dout/1
  xreg_000_dout_wr/1 -> Register3/1
  CEP3/1 -> Register3/2
  Constant3/1 -> CEP3/1
  Delay3/1 -> Data New/1
  Register3/1 -> Delay3/1
  xreg_000_dout/1 -> Register1/1
  CEP1/1 -> Register1/2
  Constant1/1 -> CEP1/1
  Delay1/1 -> Data/1
  Register1/1 -> Delay1/1

== system MG_sim/fpga/FPGA_XDATA_READ_BL2 ==
  CEP1 : xbsIndex_r4/Clock Enable Probe  inherit_constraints=off  block_type=ceprobe
      settings: infoedit="Clock enable extractor.  Produces a Boolean output that mirrors the hardware clock enable associated with the input sample rate.<br><br>Hardware notes: in hardware this block costs nothing."
  CEP3 : xbsIndex_r4/Clock Enable Probe  inherit_constraints=off  block_type=ceprobe
      settings: infoedit="Clock enable extractor.  Produces a Boolean output that mirrors the hardware clock enable associated with the input sample rate.<br><br>Hardware notes: in hardware this block costs nothing."
  Constant1 : xbsIndex_r4/Constant  const=1  gui_display_data_type=Fixed-point  arith_type=Boolean  n_bits=16  bin_pt=14  preci_type=Single  exp_width=8  frac_width=24  explicit_period=on  period=1*1e-08  equ=P=C  opselect=C  inp2=PCIN>>17  opr=+  inp1=P  carry=CIN  dbl_ovrd=off  block_type=constant
  Constant3 : xbsIndex_r4/Constant  const=1  gui_display_data_type=Fixed-point  arith_type=Boolean  n_bits=16  bin_pt=14  preci_type=Single  exp_width=8  frac_width=24  explicit_period=on  period=1*1e-08  equ=P=C  opselect=C  inp2=PCIN>>17  opr=+  inp1=P  carry=CIN  dbl_ovrd=off  block_type=constant
  Delay1 : xbsIndex_r4/Delay  rst=off  infoeditControl=Selection of Reset will increase slice count due to use of real FFs and instead of SRLs  en=off  latency=0  reg_retiming=off  dbl_ovrd=off  block_type=delay
  Delay3 : xbsIndex_r4/Delay  rst=off  infoeditControl=Selection of Reset will increase slice count due to use of real FFs and instead of SRLs  en=off  latency=0  reg_retiming=off  dbl_ovrd=off  block_type=delay
  Register1 : xbsIndex_r4/Register  init=0  rst=off  en=on  dbl_ovrd=off  block_type=register
  Register3 : xbsIndex_r4/Register  init=0  rst=off  en=on  dbl_ovrd=off  block_type=register
  phs_read_register : Subsystem
      mask init: same as MG_sim/fpga/FPGA_XDATA_READ_BL1/phs_read_register
  xreg_001_dout : xbsIndex_r4/Gateway In  gui_display_data_type=Fixed-point  arith_type=Unsigned  n_bits=32  bin_pt=0  preci_type=Single  exp_width=8  frac_width=24  rows=1  columns=1  quantization="Round  (unbiased: +/- Inf)"  overflow=Saturate  period=1e-08  UseAsADC=off  ADCChannel='1'  interface=None  automatic_assignment=on  address_offset=hex2dec('00')  intf_name=''  intf_description=''  default_value=0  timing_constraint=None  locs_specified=off  LOCs={}  io_standard={}  inherit_from_input=off  hdl_port=on  dbl_ovrd=off  block_type=gatewayin
  xreg_001_dout_wr : xbsIndex_r4/Gateway In  gui_display_data_type=Fixed-point  arith_type=Unsigned  n_bits=1  bin_pt=0  preci_type=Single  exp_width=8  frac_width=24  rows=1  columns=1  quantization="Round  (unbiased: +/- Inf)"  overflow=Saturate  period=1e-08  UseAsADC=off  ADCChannel='1'  interface=None  automatic_assignment=on  address_offset=hex2dec('00')  intf_name=''  intf_description=''  default_value=0  timing_constraint=None  locs_specified=off  LOCs={}  io_standard={}  inherit_from_input=off  hdl_port=on  dbl_ovrd=off  block_type=gatewayin
  Data : Outport
  Data New : Outport  Port=2
  wires:
  [FPGA_MG_sim_rtiFPGAtmp_1_Register_2_1_1_write] -> phs_read_register/1(data_i)
  phs_read_register/2(data_new_o) -> xreg_001_dout_wr/1
  phs_read_register/1(data_o) -> xreg_001_dout/1
  xreg_001_dout_wr/1 -> Register3/1
  CEP3/1 -> Register3/2
  Constant3/1 -> CEP3/1
  Delay3/1 -> Data New/1
  Register3/1 -> Delay3/1
  xreg_001_dout/1 -> Register1/1
  CEP1/1 -> Register1/2
  Constant1/1 -> CEP1/1
  Delay1/1 -> Data/1
  Register1/1 -> Delay1/1

== system MG_sim/fpga/FPGA_XDATA_READ_BL3 ==
  CEP1 : xbsIndex_r4/Clock Enable Probe  inherit_constraints=off  block_type=ceprobe
      settings: infoedit="Clock enable extractor.  Produces a Boolean output that mirrors the hardware clock enable associated with the input sample rate.<br><br>Hardware notes: in hardware this block costs nothing."
  CEP3 : xbsIndex_r4/Clock Enable Probe  inherit_constraints=off  block_type=ceprobe
      settings: infoedit="Clock enable extractor.  Produces a Boolean output that mirrors the hardware clock enable associated with the input sample rate.<br><br>Hardware notes: in hardware this block costs nothing."
  Constant1 : xbsIndex_r4/Constant  const=1  gui_display_data_type=Fixed-point  arith_type=Boolean  n_bits=16  bin_pt=14  preci_type=Single  exp_width=8  frac_width=24  explicit_period=on  period=1*1e-08  equ=P=C  opselect=C  inp2=PCIN>>17  opr=+  inp1=P  carry=CIN  dbl_ovrd=off  block_type=constant
  Constant3 : xbsIndex_r4/Constant  const=1  gui_display_data_type=Fixed-point  arith_type=Boolean  n_bits=16  bin_pt=14  preci_type=Single  exp_width=8  frac_width=24  explicit_period=on  period=1*1e-08  equ=P=C  opselect=C  inp2=PCIN>>17  opr=+  inp1=P  carry=CIN  dbl_ovrd=off  block_type=constant
  Delay1 : xbsIndex_r4/Delay  rst=off  infoeditControl=Selection of Reset will increase slice count due to use of real FFs and instead of SRLs  en=off  latency=0  reg_retiming=off  dbl_ovrd=off  block_type=delay
  Delay3 : xbsIndex_r4/Delay  rst=off  infoeditControl=Selection of Reset will increase slice count due to use of real FFs and instead of SRLs  en=off  latency=0  reg_retiming=off  dbl_ovrd=off  block_type=delay
  Register1 : xbsIndex_r4/Register  init=0  rst=off  en=on  dbl_ovrd=off  block_type=register
  Register3 : xbsIndex_r4/Register  init=0  rst=off  en=on  dbl_ovrd=off  block_type=register
  phs_read_register : Subsystem
      mask init: same as MG_sim/fpga/FPGA_XDATA_READ_BL1/phs_read_register
  xreg_002_dout : xbsIndex_r4/Gateway In  gui_display_data_type=Fixed-point  arith_type=Unsigned  n_bits=32  bin_pt=0  preci_type=Single  exp_width=8  frac_width=24  rows=1  columns=1  quantization="Round  (unbiased: +/- Inf)"  overflow=Saturate  period=1e-08  UseAsADC=off  ADCChannel='1'  interface=None  automatic_assignment=on  address_offset=hex2dec('00')  intf_name=''  intf_description=''  default_value=0  timing_constraint=None  locs_specified=off  LOCs={}  io_standard={}  inherit_from_input=off  hdl_port=on  dbl_ovrd=off  block_type=gatewayin
  xreg_002_dout_wr : xbsIndex_r4/Gateway In  gui_display_data_type=Fixed-point  arith_type=Unsigned  n_bits=1  bin_pt=0  preci_type=Single  exp_width=8  frac_width=24  rows=1  columns=1  quantization="Round  (unbiased: +/- Inf)"  overflow=Saturate  period=1e-08  UseAsADC=off  ADCChannel='1'  interface=None  automatic_assignment=on  address_offset=hex2dec('00')  intf_name=''  intf_description=''  default_value=0  timing_constraint=None  locs_specified=off  LOCs={}  io_standard={}  inherit_from_input=off  hdl_port=on  dbl_ovrd=off  block_type=gatewayin
  Data : Outport
  Data New : Outport  Port=2
  wires:
  [FPGA_MG_sim_rtiFPGAtmp_1_Register_3_1_1_write] -> phs_read_register/1(data_i)
  phs_read_register/2(data_new_o) -> xreg_002_dout_wr/1
  phs_read_register/1(data_o) -> xreg_002_dout/1
  xreg_002_dout_wr/1 -> Register3/1
  CEP3/1 -> Register3/2
  Constant3/1 -> CEP3/1
  Delay3/1 -> Data New/1
  Register3/1 -> Delay3/1
  xreg_002_dout/1 -> Register1/1
  CEP1/1 -> Register1/2
  Constant1/1 -> CEP1/1
  Delay1/1 -> Data/1
  Register1/1 -> Delay1/1

== system MG_sim/RTI Data/RTI Data Store/RTI Data Store ==
  RTI Data Store : Subsystem  mask(RTI_DATA_STORE){}
      mask help:
      | RTI Data Store Block. This block is used by RTI to store internal model dependent data. Deleting this block will result in data loss.
      |
      | NEVER DELETE, COPY, OR MODIFY THIS BLOCK!
      mask Help:
      | RTI Data Store Block. This block is used by RTI to store internal model dependent data. Deleting this block will result in data loss.
      | 
      | NEVER DELETE, COPY, OR MODIFY THIS BLOCK!
      mask Display: text(0.5, 0.5, ' ', 'HorizontalAlignment', 'center');

== system MG_sim/fpga/FPGA_INT_BL1/phs_interrupt ==
  note: Subsystem simulating the communication
      | function specific behaviour. This is how the
      | FPGA framework driver takes effect on the data.
  note: Subsystem simulating the phs bus
      | access via RTLib functions.
  data_i : Inport
  com_fct_model : Subsystem
  phs/rtlib_sim_model : Subsystem
  data_o : Outport  VectorParamsAs1DForOutWhenUnconnected=off
  wires:
  data_i/1 -> com_fct_model/1(data_i1)
  com_fct_model/1(data_o1) -> phs/rtlib_sim_model/1(data_i1)
  phs/rtlib_sim_model/1(data_o1) -> data_o/1

== system MG_sim/fpga/FPGA_INT_BL2/phs_interrupt ==
  note: Subsystem simulating the communication
      | function specific behaviour. This is how the
      | FPGA framework driver takes effect on the data.
  note: Subsystem simulating the phs bus
      | access via RTLib functions.
  data_i : Inport
  com_fct_model : Subsystem
  phs/rtlib_sim_model : Subsystem
  data_o : Outport  VectorParamsAs1DForOutWhenUnconnected=off
  wires:
  data_i/1 -> com_fct_model/1(data_i1)
  com_fct_model/1(data_o1) -> phs/rtlib_sim_model/1(data_i1)
  phs/rtlib_sim_model/1(data_o1) -> data_o/1

== system MG_sim/fpga/FPGA_INT_BL3/phs_interrupt ==
  note: Subsystem simulating the communication
      | function specific behaviour. This is how the
      | FPGA framework driver takes effect on the data.
  note: Subsystem simulating the phs bus
      | access via RTLib functions.
  data_i : Inport
  com_fct_model : Subsystem
  phs/rtlib_sim_model : Subsystem
  data_o : Outport  VectorParamsAs1DForOutWhenUnconnected=off
  wires:
  data_i/1 -> com_fct_model/1(data_i1)
  com_fct_model/1(data_o1) -> phs/rtlib_sim_model/1(data_i1)
  phs/rtlib_sim_model/1(data_o1) -> data_o/1

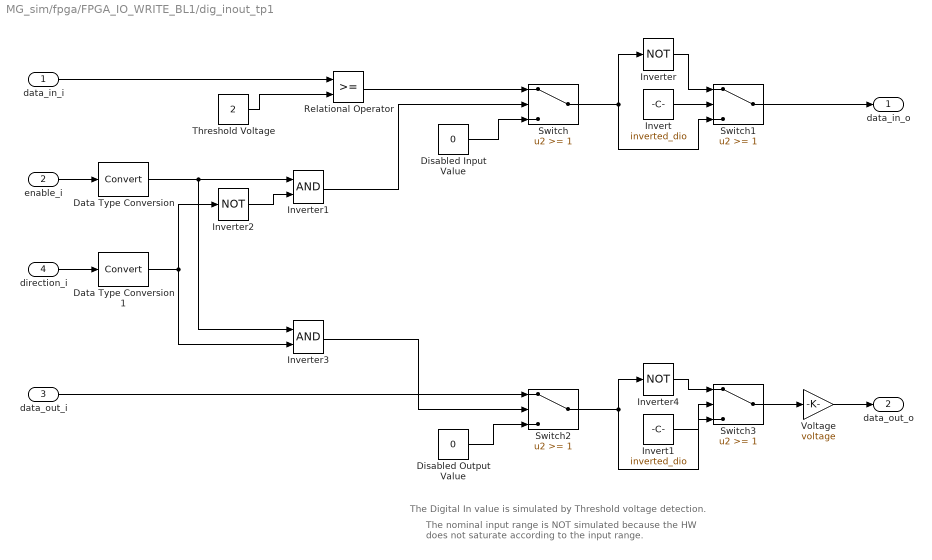
== system MG_sim/fpga/FPGA_IO_WRITE_BL1/dig_inout_tp1 ==
  note: The Digital In value is simulated by Threshold voltage detection.
  note: The nominal input range is NOT simulated because
      | the HW does not saturate according to the input range.
  data_in_i : Inport
  enable_i : Inport  Port=2
  data_out_i : Inport  Port=3
  direction_i : Inport  Port=4
  Data Type Conversion : DataTypeConversion
  Data Type Conversion1 : DataTypeConversion
  Disabled Input Value : Constant  Value=0
  Disabled Output Value : Constant  Value=0
  Invert : Constant  Value=inverted_dio
  Invert1 : Constant  Value=inverted_dio
  Inverter : Logic  Operator=NOT  AllPortsSameDT=off  OutDataTypeStr=boolean
  Inverter1 : Logic  AllPortsSameDT=off  OutDataTypeStr=boolean
  Inverter2 : Logic  Operator=NOT  AllPortsSameDT=off  OutDataTypeStr=boolean
  Inverter3 : Logic  AllPortsSameDT=off  OutDataTypeStr=boolean
  Inverter4 : Logic  Operator=NOT  AllPortsSameDT=off  OutDataTypeStr=boolean
  Relational Operator : RelationalOperator  OutDataTypeStr=boolean  RndMeth=Nearest
  Switch{,1..3} (4 alike) : Switch  Threshold=1
  Threshold Voltage : Constant  Value=2
  Voltage : Gain  Gain=voltage  ParamDataTypeStr=float('double')
  data_in_o : Outport  VectorParamsAs1DForOutWhenUnconnected=off
  data_out_o : Outport  Port=2  VectorParamsAs1DForOutWhenUnconnected=off
  wires:
  data_in_i/1 -> Relational Operator/1
  Threshold Voltage/1 -> Relational Operator/2
  Disabled Input Value/1 -> Switch/3
  Switch1/1 -> data_in_o/1
  Invert/1 -> Switch1/2
  Inverter/1 -> Switch1/1
  Relational Operator/1 -> Switch/1
  Switch/1 -> Inverter/1, Switch1/3
  enable_i/1 -> Data Type Conversion/1
  Inverter1/1 -> Switch/2
  direction_i/1 -> Data Type Conversion1/1
  Inverter2/1 -> Inverter1/2
  Disabled Output Value/1 -> Switch2/3
  Inverter3/1 -> Switch2/2
  data_out_i/1 -> Switch2/1
  Invert1/1 -> Switch3/2
  Inverter4/1 -> Switch3/1
  Switch2/1 -> Inverter4/1, Switch3/3
  Switch3/1 -> Voltage/1
  Data Type Conversion/1 -> Inverter1/1, Inverter3/1
  Data Type Conversion1/1 -> Inverter2/1, Inverter3/2
  Voltage/1 -> data_out_o/1

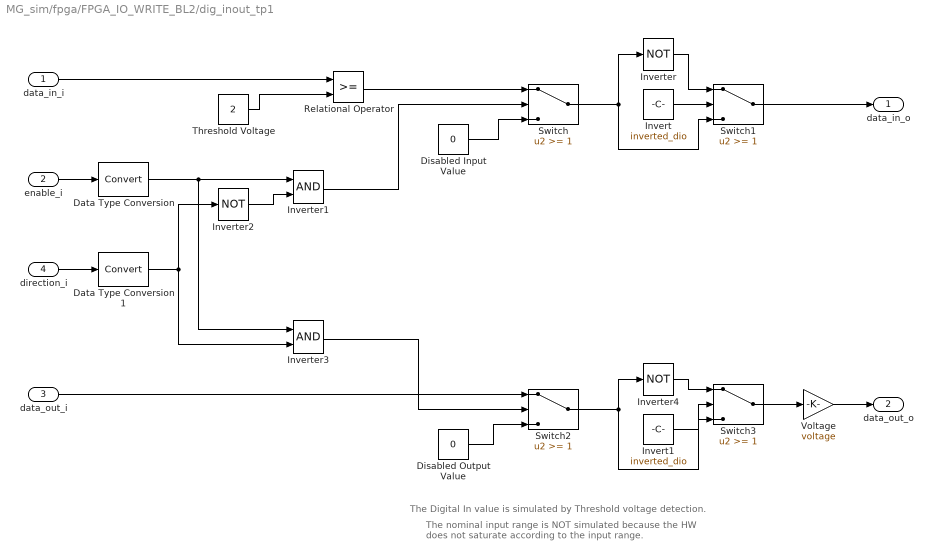
== system MG_sim/fpga/FPGA_IO_WRITE_BL2/dig_inout_tp1 ==
  note: The Digital In value is simulated by Threshold voltage detection.
  note: The nominal input range is NOT simulated because
      | the HW does not saturate according to the input range.
  data_in_i : Inport
  enable_i : Inport  Port=2
  data_out_i : Inport  Port=3
  direction_i : Inport  Port=4
  Data Type Conversion : DataTypeConversion
  Data Type Conversion1 : DataTypeConversion
  Disabled Input Value : Constant  Value=0
  Disabled Output Value : Constant  Value=0
  Invert : Constant  Value=inverted_dio
  Invert1 : Constant  Value=inverted_dio
  Inverter : Logic  Operator=NOT  AllPortsSameDT=off  OutDataTypeStr=boolean
  Inverter1 : Logic  AllPortsSameDT=off  OutDataTypeStr=boolean
  Inverter2 : Logic  Operator=NOT  AllPortsSameDT=off  OutDataTypeStr=boolean
  Inverter3 : Logic  AllPortsSameDT=off  OutDataTypeStr=boolean
  Inverter4 : Logic  Operator=NOT  AllPortsSameDT=off  OutDataTypeStr=boolean
  Relational Operator : RelationalOperator  OutDataTypeStr=boolean  RndMeth=Nearest
  Switch{,1..3} (4 alike) : Switch  Threshold=1
  Threshold Voltage : Constant  Value=2
  Voltage : Gain  Gain=voltage  ParamDataTypeStr=float('double')
  data_in_o : Outport  VectorParamsAs1DForOutWhenUnconnected=off
  data_out_o : Outport  Port=2  VectorParamsAs1DForOutWhenUnconnected=off
  wires:
  data_in_i/1 -> Relational Operator/1
  Threshold Voltage/1 -> Relational Operator/2
  Disabled Input Value/1 -> Switch/3
  Switch1/1 -> data_in_o/1
  Invert/1 -> Switch1/2
  Inverter/1 -> Switch1/1
  Relational Operator/1 -> Switch/1
  Switch/1 -> Inverter/1, Switch1/3
  enable_i/1 -> Data Type Conversion/1
  Inverter1/1 -> Switch/2
  direction_i/1 -> Data Type Conversion1/1
  Inverter2/1 -> Inverter1/2
  Disabled Output Value/1 -> Switch2/3
  Inverter3/1 -> Switch2/2
  data_out_i/1 -> Switch2/1
  Invert1/1 -> Switch3/2
  Inverter4/1 -> Switch3/1
  Switch2/1 -> Inverter4/1, Switch3/3
  Switch3/1 -> Voltage/1
  Data Type Conversion/1 -> Inverter1/1, Inverter3/1
  Data Type Conversion1/1 -> Inverter2/1, Inverter3/2
  Voltage/1 -> data_out_o/1
